simulink model "ownStateSpaceModel"  (R2015a)
settings: Solver=ode4  StartTime=0.0  StopTime=10  RelTol=1e-3
values from neighbouring files (symbols this model uses):
  A = M^(-1) * A_prim    [CreateAB.m]    (also in CreateAB2.m)
  B = M^(-1) * B_prim    [CreateAB.m]    (also in CreateAB2.m)
  x0 = [U_e; W_e; Q_e; theta_e]    [Test2.m]
undefined symbols (not defined in the file or in its folder): C, D
settings Model: Creator=adamfelis  LastModifiedBy=adamfelis

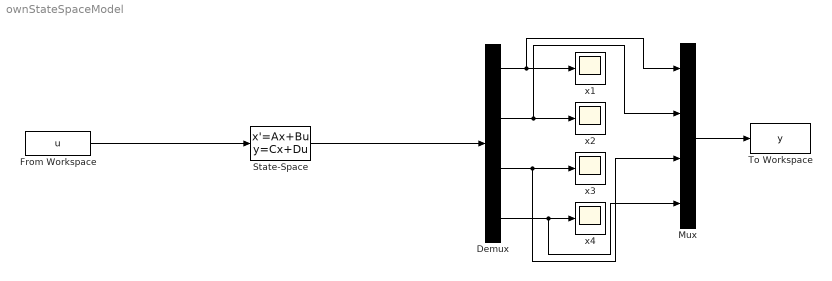
== system ownStateSpaceModel ==
  Demux : Demux
  From Workspace : FromWorkspace  VariableName=u  SampleTime=0
  Mux : Mux
  State-Space : StateSpace  A=A  B=B  C=C  D=D  X0=x0
  To Workspace : ToWorkspace  VariableName=y  SaveFormat=Timeseries  SampleTime=-1
  x{1..4} (4 alike) : Scope
      x3 settings: SaveName=ScopeData2
      x4 settings: SaveName=ScopeData4
  wires:
  State-Space/1 -> Demux/1
  Demux/4 -> Mux/4, x4/1
  Demux/2 -> Mux/2, x2/1
  Demux/1 -> Mux/1, x1/1
  Demux/3 -> Mux/3, x3/1
  Mux/1 -> To Workspace/1
  From Workspace/1 -> State-Space/1
